simulink model "prdMediumCar"  (R2023b)
settings: Solver=FixedStepDiscrete  StartTime=0.0  StopTime=100  RelTol=1e-3
settings Model: DataDictionary=prdLuxuryCar_dict.sldd  Creator=DucHM28  LastModifiedBy=DucHM28
settings OptimizationCC: DefaultParameterBehavior=Inlined  EnhancedBackFolding=on  PassReuseOutputArgsAs=Individual arguments  ZeroExternalMemoryAtStartup=off  ZeroInternalMemoryAtStartup=off  OptimizeBlockOrder=speed  DifferentSizesBufferReuse=on  OptimizationCustomize=off  EfficientTunableParamExpr=on
settings DebuggingCC: ParameterTunabilityLossMsg=error
settings SFSimCC: MATLABDynamicMemAlloc=off
settings RTWCC: Description=Embedded Coder  SystemTargetFile=ert.tlc  TemplateMakefile=ert_default_tmf  GPUComputeCapability=5.0
settings CodeAppCC: ForceParamTrailComments=on  IgnoreCustomStorageClasses=off  OperatorAnnotations=on  SimulinkDataObjDesc=on  SFDataObjDesc=on  InsertBlockDesc=on
settings ERTTargetCC: TargetLangStandard=C99 (ISO)  GenerateSampleERTMain=on  InlinedParameterPlacement=NonHierarchical  ERTCustomFileTemplate=example_file_process.tlc

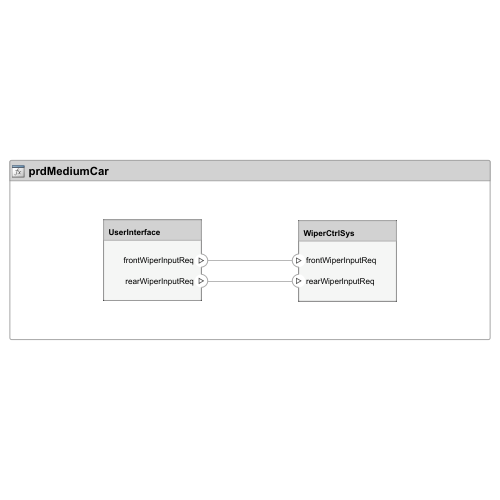
[thumbnail: Simulink's stored preview of the top-level diagram]
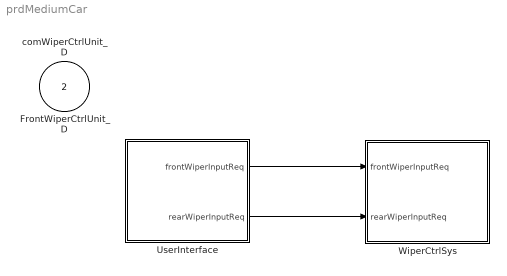
== system prdMediumCar ==
  FrontWiperCtrlUnit_D : Inport  OutputFunctionCall=on
  comWiperCtrlUnit_D : Inport  Port=2  OutputFunctionCall=on
  UserInterface : Subsystem
      settings: PortSchema="{\"entries\":[{\"content\":{\"headerSize\":26,\"margin\":15,\"minimumSpacing\":25,\"sides\":[{\"content\":{},\"type\":\"ConnectorPlacement.EquallySpacedRectSide\",\"uuid\":\"dc94f41b-7c5e-4a71-8534-53b4bbbfc770\"},{\"content\":{\"connectorIds\":[\"Out1\",\"Out2\"],\"side\":\"RIGHT\"},\"type\":\"ConnectorPlacement.EquallySpacedRectSide\",\"uuid\":\"bdf4fd69-223d-456c-8736-2799cf1eafe0\"},{\"content\":{\"side\":\"TOP\"},\"type\":\"ConnectorPlacement.EquallySpacedRectSide\",\"uuid\":\"163871d7-a199-4e1a-bbb8-d64128cdaa90\"}]},\"type\":\"ConnectorPlacement.EquallySpacedConnector\",\"uuid\":\"b4831961-b052-4c8b-b117-2d38cbc4b0c6\"}],\"packageUris\":[\"http://schema.mathworks.com/mf0/Connector/R2020b\"],\"version\":\"1.0\"}"
  WiperCtrlSys : Subsystem
      settings: PortSchema="{\"entries\":[{\"content\":{\"headerSize\":26,\"margin\":15,\"minimumSpacing\":25,\"sides\":[{\"content\":{\"connectorIds\":[\"In1\",\"In2\"]},\"type\":\"ConnectorPlacement.EquallySpacedRectSide\",\"uuid\":\"dc94f41b-7c5e-4a71-8534-53b4bbbfc770\"},{\"content\":{\"side\":\"RIGHT\"},\"type\":\"ConnectorPlacement.EquallySpacedRectSide\",\"uuid\":\"bdf4fd69-223d-456c-8736-2799cf1eafe0\"},{\"content\":{\"side\":\"TOP\"},\"type\":\"ConnectorPlacement.EquallySpacedRectSide\",\"uuid\":\"163871d7-a199-4e1a-bbb8-d64128cdaa90\"}]},\"type\":\"ConnectorPlacement.EquallySpacedConnector\",\"uuid\":\"b4831961-b052-4c8b-b117-2d38cbc4b0c6\"}],\"packageUris\":[\"http://schema.mathworks.com/mf0/Connector/R2020b\"],\"version\":\"1.0\"}"
  wires:
  UserInterface/1(frontWiperInputReq) -> WiperCtrlSys/1(frontWiperInputReq)
  UserInterface/2(rearWiperInputReq) -> WiperCtrlSys/2(rearWiperInputReq)

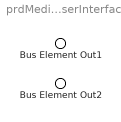
== system prdMediumCar/UserInterface ==
  Bus Element Out1 : Outport  AllowServiceAccess=on  PortName=frontWiperInputReq
  Bus Element Out2 : Outport  Port=2  AllowServiceAccess=on  PortName=rearWiperInputReq

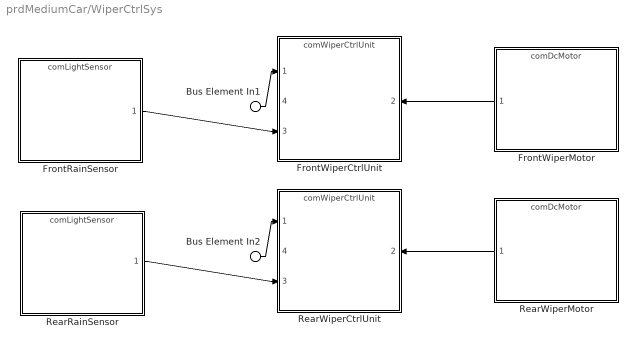
== system prdMediumCar/WiperCtrlSys ==
  Bus Element In1 : Inport  AllowServiceAccess=on  PortName=frontWiperInputReq
  Bus Element In2 : Inport  Port=2  AllowServiceAccess=on  PortName=rearWiperInputReq
  FrontRainSensor : ModelReference  ModelNameDialog=comLightSensor  SimulationMode=Normal  ScheduleRates=on  ModelReferenceVersion=1.29
      settings: PortSchema="{\"entries\":[{\"content\":{\"headerSize\":38,\"margin\":15,\"minimumSpacing\":25,\"sides\":[{\"content\":{},\"type\":\"ConnectorPlacement.EquallySpacedRectSide\",\"uuid\":\"dc94f41b-7c5e-4a71-8534-53b4bbbfc770\"},{\"content\":{\"connectorIds\":[\"Out1\"],\"side\":\"RIGHT\"},\"type\":\"ConnectorPlacement.EquallySpacedRectSide\",\"uuid\":\"bdf4fd69-223d-456c-8736-2799cf1eafe0\"},{\"content\":{\"side\":\"TOP\"},\"type\":\"ConnectorPlacement.EquallySpacedRectSide\",\"uuid\":\"163871d7-a199-4e1a-bbb8-d64128cdaa90\"},{\"content\":{\"side\":\"BOTTOM\"},\"type\":\"ConnectorPlacement.EquallySpacedRectSide\",\"uuid\":\"f971a296-6dad-49db-a7ca-1dd16380e6f4\"},{\"content\":{\"side\":\"HIDDEN\"},\"type\":\"ConnectorPlacement.EquallySpacedRectSide\",\"uuid\":\"10867e30-f888-4c21-b4a2-e9a2a5833dde\"}]},\"type\":\"ConnectorPlacement.EquallySpacedConnector\",\"uuid\":\"b4831961-b052-4c8b-b117-2d38cbc4b0c6\"}],\"packageUris\":[\"http://schema.mathworks.com/mf0/Connector/R2020b\"],\"version\":\"1.0\"}"
  FrontWiperCtrlUnit : ModelReference  ModelNameDialog=comWiperCtrlUnit  UsingDefaultArgumentValue=0,0,0,0  SimulationMode=Normal  ScheduleRates=on  CachedPortDiscreteRates=[-1]  ModelReferenceVersion=1.36
      settings: PortSchema="{\"entries\":[{\"content\":{\"headerSize\":38,\"margin\":15,\"minimumSpacing\":25,\"sides\":[{\"content\":{\"connectorIds\":[\"In1\",\"In3\"]},\"type\":\"ConnectorPlacement.EquallySpacedRectSide\",\"uuid\":\"dc94f41b-7c5e-4a71-8534-53b4bbbfc770\"},{\"content\":{\"connectorIds\":[\"In2\"],\"side\":\"RIGHT\"},\"type\":\"ConnectorPlacement.EquallySpacedRectSide\",\"uuid\":\"bdf4fd69-223d-456c-8736-2799cf1eafe0\"},{\"content\":{\"side\":\"TOP\"},\"type\":\"ConnectorPlacement.EquallySpacedRectSide\",\"uuid\":\"163871d7-a199-4e1a-bbb8-d64128cdaa90\"},{\"content\":{\"side\":\"BOTTOM\"},\"type\":\"ConnectorPlacement.EquallySpacedRectSide\",\"uuid\":\"ad39bc48-8c2f-4675-8e27-e9bebcc39a94\"},{\"content\":{\"connectorIds\":[\"In4\"],\"side\":\"HIDDEN\"},\"type\":\"ConnectorPlacement.EquallySpacedRectSide\",\"uuid\":\"b5f37a8d-1196-437b-803c-fa4e54e5886a\"}]},\"type\":\"ConnectorPlacement.EquallySpacedConnector\",\"uuid\":\"b4831961-b052-4c8b-b117-2d38cbc4b0c6\"}],\"packageUris\":[\"http://schema.mathworks.com/mf0/Connector/R2020b\"],\"version\":\"1.0\"}"
  FrontWiperMotor : ModelReference  ModelNameDialog=comDcMotor  SimulationMode=Normal  ScheduleRates=on  ModelReferenceVersion=1.31
      settings: PortSchema="{\"entries\":[{\"content\":{\"headerSize\":38,\"margin\":15,\"minimumSpacing\":25,\"sides\":[{\"content\":{\"connectorIds\":[\"Out1\"]},\"type\":\"ConnectorPlacement.EquallySpacedRectSide\",\"uuid\":\"dc94f41b-7c5e-4a71-8534-53b4bbbfc770\"},{\"content\":{\"side\":\"RIGHT\"},\"type\":\"ConnectorPlacement.EquallySpacedRectSide\",\"uuid\":\"bdf4fd69-223d-456c-8736-2799cf1eafe0\"},{\"content\":{\"side\":\"TOP\"},\"type\":\"ConnectorPlacement.EquallySpacedRectSide\",\"uuid\":\"163871d7-a199-4e1a-bbb8-d64128cdaa90\"}]},\"type\":\"ConnectorPlacement.EquallySpacedConnector\",\"uuid\":\"b4831961-b052-4c8b-b117-2d38cbc4b0c6\"}],\"packageUris\":[\"http://schema.mathworks.com/mf0/Connector/R2020b\"],\"version\":\"1.0\"}"
  RearRainSensor : ModelReference  ModelNameDialog=comLightSensor.slx  SimulationMode=Normal  ScheduleRates=on  ModelReferenceVersion=1.29
      settings: PortSchema="{\"entries\":[{\"content\":{\"headerSize\":38,\"margin\":15,\"minimumSpacing\":25,\"sides\":[{\"content\":{},\"type\":\"ConnectorPlacement.EquallySpacedRectSide\",\"uuid\":\"29178085-c466-4563-9f85-ead00d2b8fe4\"},{\"content\":{\"connectorIds\":[\"Out1\"],\"side\":\"RIGHT\"},\"type\":\"ConnectorPlacement.EquallySpacedRectSide\",\"uuid\":\"aa440289-fbe2-4462-afb3-1ddac7def83f\"},{\"content\":{\"side\":\"TOP\"},\"type\":\"ConnectorPlacement.EquallySpacedRectSide\",\"uuid\":\"67d32b8d-46ec-409e-8fd1-97c1fafd177c\"}]},\"type\":\"ConnectorPlacement.EquallySpacedConnector\",\"uuid\":\"11530947-54d2-4e6a-bf82-7117d3bc50c0\"}],\"packageUris\":[\"http://schema.mathworks.com/mf0/Connector/R2020b\"],\"version\":\"1.0\"}"
  RearWiperCtrlUnit : ModelReference  ModelNameDialog=comWiperCtrlUnit.slx  UsingDefaultArgumentValue=0,0,0,0  SimulationMode=Normal  ScheduleRates=on  CachedPortDiscreteRates=[-1]  ModelReferenceVersion=1.36
      settings: PortSchema="{\"entries\":[{\"content\":{\"headerSize\":38,\"margin\":15,\"minimumSpacing\":25,\"sides\":[{\"content\":{\"connectorIds\":[\"In1\",\"In3\"]},\"type\":\"ConnectorPlacement.EquallySpacedRectSide\",\"uuid\":\"75e5bac0-749d-43ad-861e-ba73e74c49b3\"},{\"content\":{\"connectorIds\":[\"In2\"],\"side\":\"RIGHT\"},\"type\":\"ConnectorPlacement.EquallySpacedRectSide\",\"uuid\":\"0bf3d68b-8056-4927-afd6-7dd5186ac4e9\"},{\"content\":{\"side\":\"TOP\"},\"type\":\"ConnectorPlacement.EquallySpacedRectSide\",\"uuid\":\"1e44d080-7fea-4d02-a485-a67784d10c1e\"},{\"content\":{\"connectorIds\":[\"In4\"],\"side\":\"HIDDEN\"},\"type\":\"ConnectorPlacement.EquallySpacedRectSide\",\"uuid\":\"d25803ca-e995-46c4-917f-5be8bedf237c\"}]},\"type\":\"ConnectorPlacement.EquallySpacedConnector\",\"uuid\":\"bd897e1c-2536-4aff-b481-f4b25bcb0dc6\"}],\"packageUris\":[\"http://schema.mathworks.com/mf0/Connector/R2020b\"],\"version\":\"1.0\"}"
  RearWiperMotor : ModelReference  ModelNameDialog=comDcMotor.slx  SimulationMode=Normal  ScheduleRates=on  ModelReferenceVersion=1.31
      settings: PortSchema="{\"entries\":[{\"content\":{\"headerSize\":38,\"margin\":15,\"minimumSpacing\":25,\"sides\":[{\"content\":{\"connectorIds\":[\"Out1\"]},\"type\":\"ConnectorPlacement.EquallySpacedRectSide\",\"uuid\":\"321da595-8ff5-4a44-b2e8-2e6f280b2cb2\"},{\"content\":{\"side\":\"RIGHT\"},\"type\":\"ConnectorPlacement.EquallySpacedRectSide\",\"uuid\":\"577632e8-f448-4077-a9bb-ef78192d9e62\"},{\"content\":{\"side\":\"TOP\"},\"type\":\"ConnectorPlacement.EquallySpacedRectSide\",\"uuid\":\"cb878c1f-59a1-4128-825f-8448de380d7d\"}]},\"type\":\"ConnectorPlacement.EquallySpacedConnector\",\"uuid\":\"54c6ce09-89ac-4374-b60b-cf7e21a31667\"}],\"packageUris\":[\"http://schema.mathworks.com/mf0/Connector/R2020b\"],\"version\":\"1.0\"}"
  wires:
  Bus Element In1/1 -> FrontWiperCtrlUnit/1
  FrontRainSensor/1 -> FrontWiperCtrlUnit/3
  RearWiperMotor/1 -> RearWiperCtrlUnit/2
  Bus Element In2/1 -> RearWiperCtrlUnit/1
  RearRainSensor/1 -> RearWiperCtrlUnit/3
  FrontWiperMotor/1 -> FrontWiperCtrlUnit/2
